simulink model "geo_affine"  (Simulink 10.2)
settings: Solver=FixedStepDiscrete  StartTime=0.0  StopTime=0  RelTol=1e-3  EnableMultiTasking=on
undefined symbols (not defined in the file or in its folder): gray
libraries: visionsources x1, visiongeotforms x1
settings Model: Creator=FxMain  LastModifiedBy=Vasil
settings DataIOCC: LimitDataPoints=on
settings OptimizationCC: ExpressionDepthLimit=2147483647
settings DebuggingCC: SolverPrmCheckMsg=warning  StateNameClashWarn=warning
settings ConfigComp: CovExternalEMLEnable=on

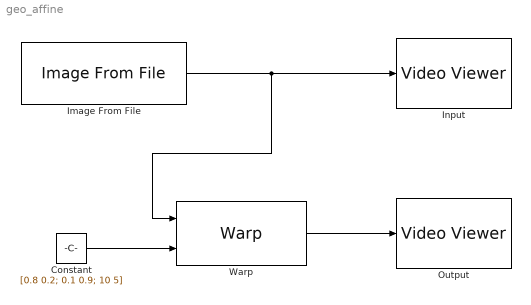
== system geo_affine ==
  Constant : Constant  Value=[0.8 0.2; 0.1 0.9; 10 5]  VectorParams1D=off
      settings: SamplingMode=Frame based
  Image From File : visionsources/Image From File  Tag=vipblks_nd  FileName=peppers.png  Ts=inf  imagePorts=One multidimensional signal  OutPortLabels=R|G|B  ImageDataType=Inherit from input image  sdImageDataType=uint(8)  Signed=on  WordLength=16  FractionLengthMode=User-defined  FractionLength=15
  Input : VideoViewer  FigPos=[75.4 490.8 417.6 304]
  Output : VideoViewer  colormapValue=gray(256)  FigPos=[493 514 417.6 304]
  Warp : visiongeotforms/Warp  TransformMatrixSource=Input port  TransformMatrix=eye( 3 )  InterpolationMethod=Bicubic  BackgroundFillValue=0  OutputImagePositionSource=Same as input image  OutputImagePosition=[ 1, 1, 512, 512 ]  ROIInputPort=off  ROIValidityOutputPort=off  SimulateUsing=Interpreted execution
      settings: SourceProductBaseCode=VP
  wires:
  Image From File/1 -> Warp/1, Input/1
  Warp/1 -> Output/1
  Constant/1 -> Warp/2
